simulink model "main"  (R2022a)
settings: Solver=VariableStepAuto  StartTime=0.0  StopTime=10  FixedStep=Ts  RelTol=1e-3
undefined symbols (not defined in the file): phi_ref, psi_ref, theta_ref, z_ref
settings Model: Creator=juani  LastModifiedBy=juani
settings SolverCC: ZeroCrossAlgorithm=Adaptive
settings DataIOCC: Refine=100
settings DebuggingCC: IgnoredZcDiagnostic=none
settings ModelReferenceCC: ModelReferenceMinAlgLoopOccurrences=on

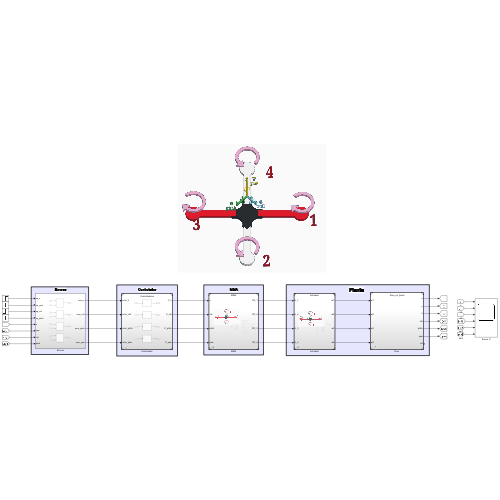
[thumbnail: Simulink's stored preview of the top-level diagram]
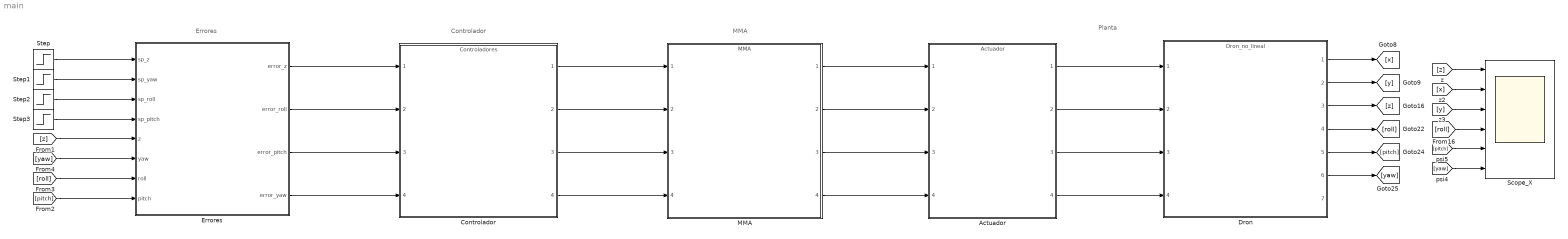
== system main ==
  note: Planta
  note: Controlador
  note: Errores
  note: MMA
  Actuador : ModelReference  ModelNameDialog=Actuador.slx  SimulationMode=Normal  ModelReferenceVersion=1.14
  Controlador : ModelReference  ModelNameDialog=Controladores.slx  SimulationMode=Normal  ModelReferenceVersion=1.14
  Dron : ModelReference  ModelNameDialog=Dron_no_lineal.slx  SimulationMode=Normal  ModelReferenceVersion=1.137
  Errores : Subsystem
  MMA : ModelReference  ModelNameDialog=MMA.slx  SimulationMode=Normal  ModelReferenceVersion=1.28
  Scope_X : Scope  NumInputPorts=6
  Step : Step  Time=0.2  After=z_ref  SampleTime=0
  Step1 : Step  Time=0.2  After=psi_ref  SampleTime=0
  Step2 : Step  Time=0.2  After=phi_ref  SampleTime=0
  Step3 : Step  Time=0.2  After=theta_ref  SampleTime=0
  wires:
  [z] -> Scope_X/1
  Controlador/1 -> MMA/1
  [roll] -> Scope_X/4
  [pitch] -> Scope_X/5
  [x] -> Scope_X/2
  [y] -> Scope_X/3
  [yaw] -> Scope_X/6
  Dron/2 -> [y]
  Dron/6 -> [yaw]
  Dron/3 -> [z]
  Dron/1 -> [x]
  Dron/5 -> [pitch]
  Dron/4 -> [roll]
  Errores/1(error_z) -> Controlador/1
  MMA/1 -> Actuador/1
  MMA/2 -> Actuador/2
  MMA/3 -> Actuador/3
  MMA/4 -> Actuador/4
  Actuador/1 -> Dron/1
  Actuador/2 -> Dron/2
  Actuador/4 -> Dron/4
  Actuador/3 -> Dron/3
  Step/1 -> Errores/1(sp_z)
  Step1/1 -> Errores/2(sp_yaw)
  Step2/1 -> Errores/3(sp_roll)
  Step3/1 -> Errores/4(sp_pitch)
  [z] -> Errores/5(z)
  [pitch] -> Errores/8(pitch)
  [roll] -> Errores/7(roll)
  [yaw] -> Errores/6(yaw)
  Errores/2(error_roll) -> Controlador/2
  Errores/3(error_pitch) -> Controlador/3
  Errores/4(error_yaw) -> Controlador/4
  Controlador/3 -> MMA/3
  Controlador/2 -> MMA/2
  Controlador/4 -> MMA/4

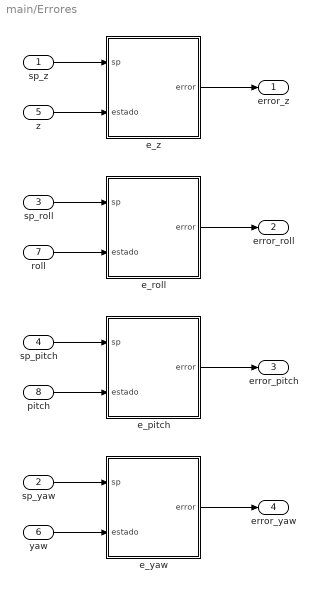
== system main/Errores ==
  sp_z : Inport
  sp_yaw : Inport  Port=2
  sp_roll : Inport  Port=3
  sp_pitch : Inport  Port=4
  z : Inport  Port=5
  yaw : Inport  Port=6
  roll : Inport  Port=7
  pitch : Inport  Port=8
  e_pitch : Subsystem
  e_roll : Subsystem
  e_yaw : Subsystem
  e_z : Subsystem
  error_z : Outport
  error_roll : Outport  Port=2
  error_pitch : Outport  Port=3
  error_yaw : Outport  Port=4
  wires:
  sp_z/1 -> e_z/1(sp)
  sp_yaw/1 -> e_yaw/1(sp)
  sp_pitch/1 -> e_pitch/1(sp)
  sp_roll/1 -> e_roll/1(sp)
  z/1 -> e_z/2(estado)
  yaw/1 -> e_yaw/2(estado)
  roll/1 -> e_roll/2(estado)
  pitch/1 -> e_pitch/2(estado)
  e_z/1(error) -> error_z/1
  e_yaw/1(error) -> error_yaw/1
  e_pitch/1(error) -> error_pitch/1
  e_roll/1(error) -> error_roll/1

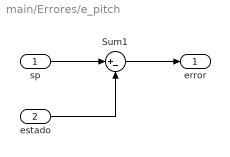
== system main/Errores/e_pitch ==
  sp : Inport
  estado : Inport  Port=2
  Sum1 : Sum  Inputs=|+-
  error : Outport
  wires:
  sp/1 -> Sum1/1
  Sum1/1 -> error/1
  estado/1 -> Sum1/2

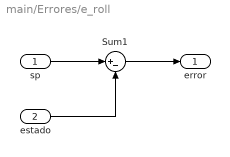
== system main/Errores/e_roll ==
  sp : Inport
  estado : Inport  Port=2
  Sum1 : Sum  Inputs=|+-
  error : Outport
  wires:
  sp/1 -> Sum1/1
  Sum1/1 -> error/1
  estado/1 -> Sum1/2

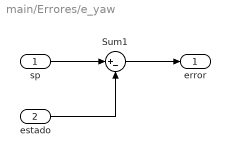
== system main/Errores/e_yaw ==
  sp : Inport
  estado : Inport  Port=2
  Sum1 : Sum  Inputs=|+-
  error : Outport
  wires:
  sp/1 -> Sum1/1
  Sum1/1 -> error/1
  estado/1 -> Sum1/2

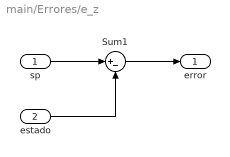
== system main/Errores/e_z ==
  sp : Inport
  estado : Inport  Port=2
  Sum1 : Sum  Inputs=|+-
  error : Outport
  wires:
  sp/1 -> Sum1/1
  Sum1/1 -> error/1
  estado/1 -> Sum1/2
